simulink model "Aeropendulum_new_model_v2"  (R2021b)
settings: Solver=VariableStepAuto  StartTime=0.0  StopTime=10  RelTol=1e-3
values from neighbouring files (symbols this model uses):
  c = 0.007    [ANM_params.m]    (also in ANM_params_test.m)
  d = 0.25    [ANM_params.m]    (also in ANM_params_test.m)
  g = 9.81    [ANM_params.m]    (also in ANM_params_test.m)
  J = m*l*l    (= 0.0075)    [ANM_params.m]    (also in ANM_params_test.m)
  l = 0.25    [ANM_params.m]    (also in ANM_params_test.m)
  m = 0.120    (= 0.12)    [ANM_params.m]    (also in ANM_params_test.m)
  Rs = 5    [ANM_params.m]
  Ts = 0.01    [ANM_DDPG_agent.m]    (also in ANM_params.m; ANM_params_test.m)
  yref = 30    [ANM_params.m]    (also in ANM_params_test.m = 25; ANM_train_loop.m = 20)
libraries: rllib x1, simulink x1
settings Model: Creator=Marcin  LastModifiedBy=Marcin

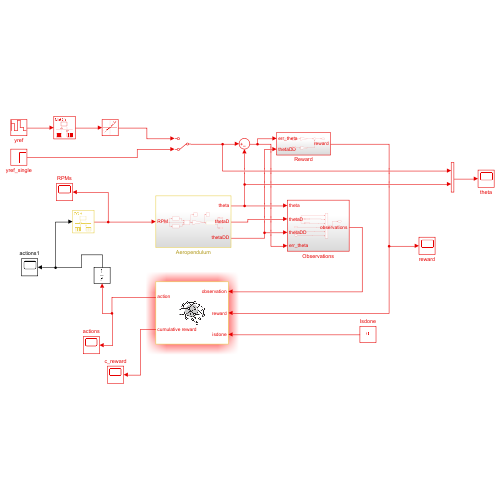
[thumbnail: Simulink's stored preview of the top-level diagram]
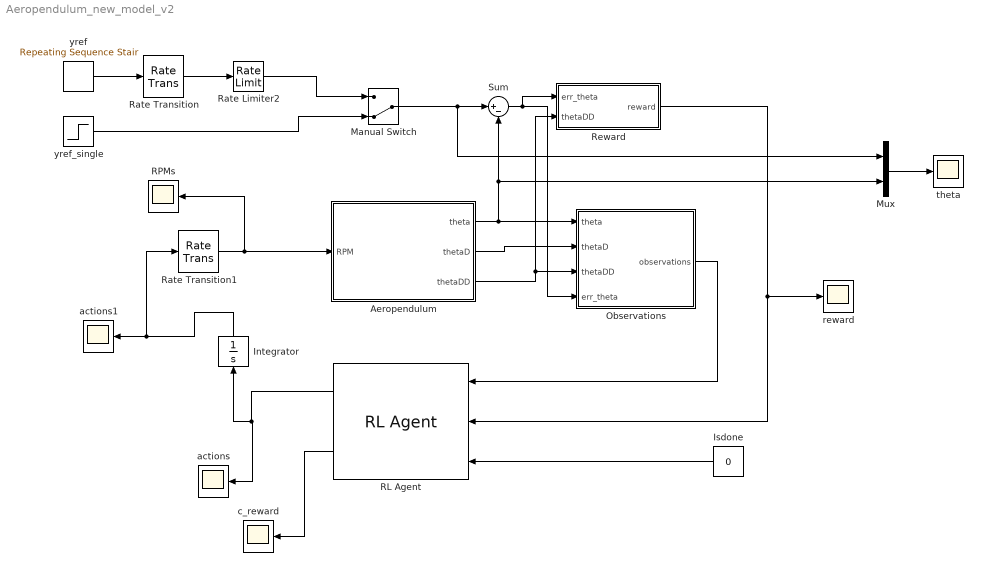
== system Aeropendulum_new_model_v2 ==
  Aeropendulum : Subsystem
  Integrator : Integrator
  Isdone : Constant  Value=0  SampleTime=Ts
  Manual Switch : ManualSwitch  CurrentSetting=0
  Mux : Mux  Inputs=2
  Observations : Subsystem
  RL Agent : rllib/RL Agent  Agent=saved_agent  ExternalActionAsInput=off  ProvideCumRwd=on  TreatAsDirectFeedthrough=on
  RPMs : Scope
  Rate Limiter2 : RateLimiter  RisingSlewLimit=Rs  FallingSlewLimit=-Rs  SampleTimeMode=inherited
  Rate Transition : RateTransition  InitialCondition=10  OutPortSampleTime=Ts
  Rate Transition1 : RateTransition  OutPortSampleTime=Ts
  Reward : Subsystem
  Sum : Sum  Inputs=|+-
  actions : Scope
  actions1 : Scope
  c_reward : Scope
  reward : Scope
  theta : Scope
  yref : simulink/Sources/Repeating Sequence Stair  OutValues=input_yref_vector  tsamp=Ts  OutMin=[]  OutMax=[]  OutDataTypeStr=double  OutputDataTypeScalingMode=double  OutDataType=fixdt(0,8)  ConRadixGroup=Best Precision: Vector-wise  OutScaling=2^-12
  yref_single : Step  Time=0  After=yref  SampleTime=Ts
  wires:
  Aeropendulum/2(thetaD) -> Observations/2(thetaD)
  Aeropendulum/3(thetaDD) -> Reward/2(thetaDD), Observations/3(thetaDD)
  Observations/1(observations) -> RL Agent/1
  Aeropendulum/1(theta) -> Sum/2, Mux/2, Observations/1(theta)
  Reward/1(reward) -> reward/1, RL Agent/2
  Mux/1 -> theta/1
  Manual Switch/1 -> Mux/1, Sum/1
  Isdone/1 -> RL Agent/3
  Sum/1 -> Observations/4(err_theta), Reward/1(err_theta)
  Rate Transition/1 -> Rate Limiter2/1
  yref/1 -> Rate Transition/1
  Rate Limiter2/1 -> Manual Switch/1
  yref_single/1 -> Manual Switch/2
  RL Agent/1 -> Integrator/1, actions/1
  Rate Transition1/1 -> Aeropendulum/1(RPM), RPMs/1
  Integrator/1 -> Rate Transition1/1, actions1/1
  RL Agent/2 -> c_reward/1

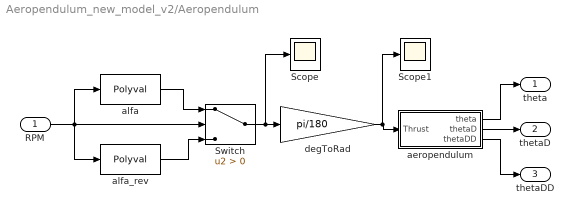
== system Aeropendulum_new_model_v2/Aeropendulum ==
  RPM : Inport
  Scope : Scope
  Scope1 : Scope
  Switch : Switch  Criteria=u2 > Threshold
  aeropendulum : Subsystem
  alfa : Polyval  Coefs="[3.04986021927422e-06,  -0.00476887717971010 , 2.51670431281220]"
  alfa_rev : Polyval  Coefs="[-5.46944010985214e-06,\t-0.00938361577873603,\t-2.43262552689868]"
  degToRad : Gain  Gain=pi/180
  theta : Outport
  thetaD : Outport  Port=2
  thetaDD : Outport  Port=3
  wires:
  alfa/1 -> Switch/1
  RPM/1 -> alfa_rev/1, alfa/1, Switch/2
  Switch/1 -> Scope/1, degToRad/1
  degToRad/1 -> Scope1/1, aeropendulum/1(Thrust)
  alfa_rev/1 -> Switch/3
  aeropendulum/1(theta) -> theta/1
  aeropendulum/2(thetaD) -> thetaD/1
  aeropendulum/3(thetaDD) -> thetaDD/1

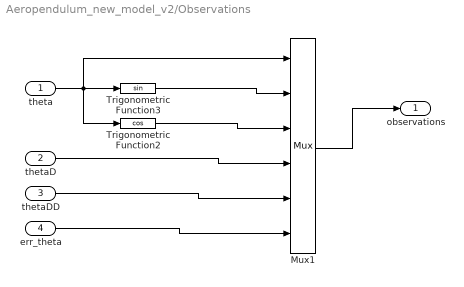
== system Aeropendulum_new_model_v2/Observations ==
  theta : Inport
  thetaD : Inport  Port=2
  thetaDD : Inport  Port=3
  err_theta : Inport  Port=4
  Mux1 : Mux  Inputs=6
  Trigonometric Function2 : Trigonometry  Operator=cos
  Trigonometric Function3 : Trigonometry
  observations : Outport
  wires:
  theta/1 -> Mux1/1, Trigonometric Function3/1, Trigonometric Function2/1
  Mux1/1 -> observations/1
  err_theta/1 -> Mux1/6
  thetaDD/1 -> Mux1/5
  thetaD/1 -> Mux1/4
  Trigonometric Function2/1 -> Mux1/3
  Trigonometric Function3/1 -> Mux1/2

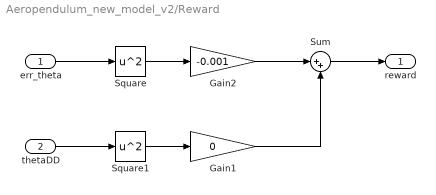
== system Aeropendulum_new_model_v2/Reward ==
  err_theta : Inport
  thetaDD : Inport  Port=2
  Gain1 : Gain  Gain=0
  Gain2 : Gain  Gain=-0.001
  Square : Math  Operator=square  SaturateOnIntegerOverflow=on
  Square1 : Math  Operator=square  SaturateOnIntegerOverflow=on
  Sum : Sum  Inputs=|++
  reward : Outport
  wires:
  err_theta/1 -> Square/1
  Square/1 -> Gain2/1
  thetaDD/1 -> Square1/1
  Square1/1 -> Gain1/1
  Sum/1 -> reward/1
  Gain2/1 -> Sum/1
  Gain1/1 -> Sum/2

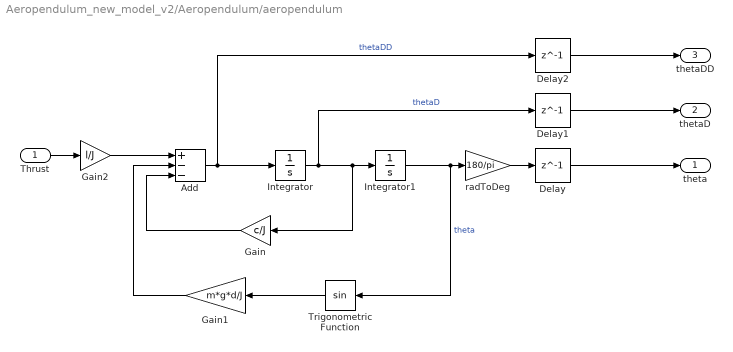
== system Aeropendulum_new_model_v2/Aeropendulum/aeropendulum ==
  Thrust : Inport
  Add : Sum  Inputs=+--
  Delay : Delay  DelayLength=1  InitialCondition=0
  Delay1 : Delay  DelayLength=1  InitialCondition=0
  Delay2 : Delay  DelayLength=1  InitialCondition=0
  Gain : Gain  Gain=c/J
  Gain1 : Gain  Gain=m*g*d/J
  Gain2 : Gain  Gain=l/J
  Integrator : Integrator
  Integrator1 : Integrator
  Trigonometric Function : Trigonometry
  radToDeg : Gain  Gain=180/pi
  theta : Outport
  thetaD : Outport  Port=2
  thetaDD : Outport  Port=3
  wires:
  Thrust/1 -> Gain2/1
  Integrator/1 -> Delay1/1, Gain/1, Integrator1/1  "thetaD"
  Integrator1/1 -> Trigonometric Function/1, radToDeg/1  "theta"
  Add/1 -> Delay2/1, Integrator/1  "thetaDD"
  Gain1/1 -> Add/2
  Trigonometric Function/1 -> Gain1/1
  Gain/1 -> Add/3
  Gain2/1 -> Add/1
  radToDeg/1 -> Delay/1
  Delay1/1 -> thetaD/1
  Delay2/1 -> thetaDD/1
  Delay/1 -> theta/1
